simulink model "RCcasestudy"  (R2020a)
settings: Solver=VariableStepAuto  StartTime=0.0  StopTime=T  FixedStep=0  RelTol=1e-3
InitFcn:
  | run init.m
values from neighbouring files (symbols this model uses):
  C = 1e-2    (= 0.01)    [RCcasestudyscriptSample.m]    (also in init.m = 2e-06)
  C_1 = 2e-7    (= 2e-07)    [RCcasestudyscriptSample.m]    (also in init.m)
  C_2 = 2e-6    (= 2e-06)    [RCcasestudyscriptSample.m]    (also in init.m)
  R = 1000    [RCcasestudyscriptSample.m]    (also in init.m)
  R_1 = 320    [RCcasestudyscriptSample.m]    (also in init.m)
  R_2 = 400    [RCcasestudyscriptSample.m]    (also in init.m)
undefined symbols (not defined in the file or in its folder): Fs
libraries: slctrlblks x3
settings Model: Creator=ethan  LastModifiedBy=ethan
settings DataIOCC: ReturnWorkspaceOutputsName=simdata

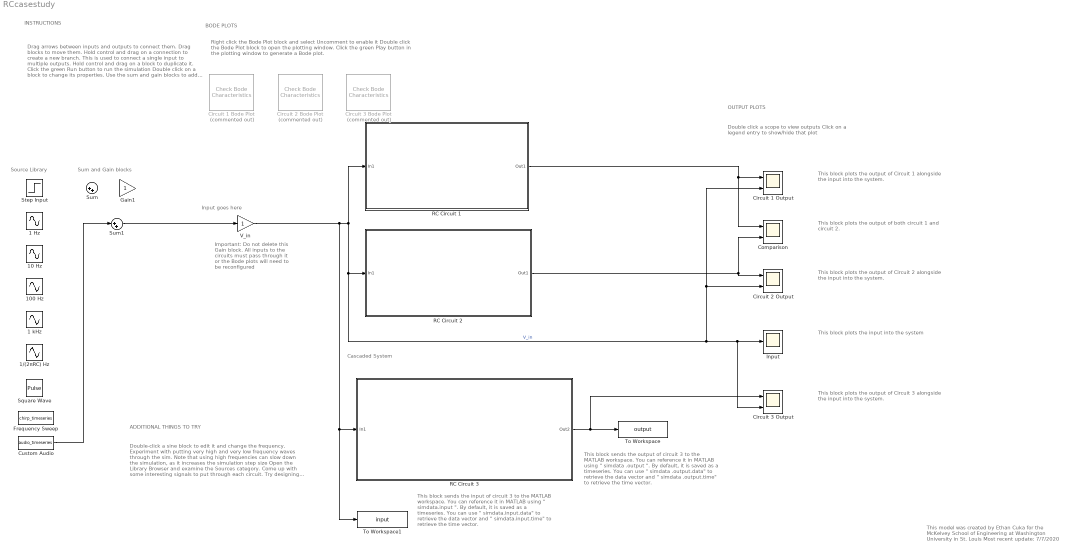
== system RCcasestudy ==
  note: This model was created by Ethan Cuka for the McKelvey School of Engineering at Washington University in St. Louis
      | Most recent update: 7/7/2020
  note: Double click a scope to view outputs
      |
      | Click on a legend entry to show/hide that plot
  note: Cascaded System
  note: Input goes here
  note: Sum and Gain blocks
  note: INSTRUCTIONS
  note: Source Library
  note: Important: Do not delete this Gain block. All inputs to the circuits must pass through it or the Bode plots will need to be reconfigured
  note: Right click the Bode Plot block and select Uncomment to enable it
      |
      | Double click the Bode Plot block to open the plotting window.
      |
      | Click the green Play button in the plotting window to generate a Bode plot.
  note: Drag arrows between inputs and outputs to connect them. Drag blocks to move them.
      |
      | Hold control and drag on a connection to create a new branch. This is used to connect a single input to multiple outputs. Hold control and drag on a block to duplicate it.
      |
      | Click the green Run button to run the simulation
      |
      | Double click on a block to change its properties.
      |
      | Use the sum and gain blocks to add combinations of waveforms together to create a superposition. Explore what happens to superimposed signals as they pass through each circuit.
  note: BODE PLOTS
  note: OUTPUT PLOTS
  note: This block plots the output of Circuit 1 alongside the input into the system.
  note: This block plots the output of both circuit 1 and circuit 2.
  note: This block plots the output of Circuit 2 alongside the input into the system.
  note: This block plots the input into the system
  note: This block plots the output of Circuit 3 alongside the input into the system.
  note: This block sends the output of circuit 3 to the MATLAB workspace. You can reference it in MATLAB using " simdata .output ". By default, it is saved as a timeseries. You can use " simdata .output.data" to retrieve the data vector and " simdata .output.time" to retrieve the time vector.
  note: ADDITIONAL THINGS TO TRY
  note: Double-click a sine block to edit it and change the frequency. Experiment with putting very high and very low frequency waves through the sim. Note that using high frequencies can slow down the simulation, as it increases the simulation step size
      |
      | Open the Library Browser and examine the Sources category. Come up with some interesting signals to put through each circuit.
      |
      | Try designing your own circuit to test. The simplest implementation in Simulink is to find the transfer function of your circuit and use the Transfer Function block.
  note: This block sends the input of circuit 3 to the MATLAB workspace. You can reference it in MATLAB using " simdata.input ". By default, it is saved as a timeseries. You can use " simdata.input.data" to retrieve the data vector and " simdata.input.time" to retrieve the time vector.
  1 Hz : Sin  Frequency=2*pi  SampleTime=0
  1 kHz : Sin  Frequency=2*pi*1000  SampleTime=0
  1/(2πRC) Hz : Sin  Frequency=1/(R*C)  SampleTime=0
  10 Hz : Sin  Frequency=2*pi*10  SampleTime=0
  100 Hz : Sin  Frequency=2*pi*100  SampleTime=0
  Circuit 1 Bode Plot : slctrlblks/Model Verification/Check Bode  Characteristics  Commented=on  InstantiateOnLoad=on  SaveOperatingPoints=off  LinearizationIOs={'/RC Circuit 1', 1, 'out', 'on', '';'/V_in', 1, 'in', 'off', ''}  LinearizeAt=SnapshotTimes  SnapshotTimes=[0]  TriggerType=rising  SampleTime=auto  RateConversionMethod=zoh  PreWarpFreq=10  UseExactDelayModel=off  UseFullBlockNameLabels=off  UseBusSignalLabels=off  enabled=on  stopWhenAssertionFail=off  export=off  ViewDlgPos=[-2.2 145 764.8 518.4]  OpenViewOnLoad=on  LaunchViewOnOpen=on  FrequencyUnits=rad/s  MagnitudeUnits=dB  PhaseUnits=deg  TimeUnits=seconds  EnableUpperBound=off  UpperBoundFrequencies=[]  UpperBoundMagnitudes=[]  EnableLowerBound=off  LowerBoundFrequencies=[]  LowerBoundMagnitudes=[]
      settings: SaveToWorkspace=on  SaveName=bode
  Circuit 1 Output : Scope  NumInputPorts=2
  Circuit 2 Bode Plot : slctrlblks/Model Verification/Check Bode  Characteristics  Commented=on  InstantiateOnLoad=on  SaveOperatingPoints=off  LinearizationIOs={'/RC Circuit 2', 1, 'out', 'on', '';'/V_in', 1, 'in', 'off', ''}  LinearizeAt=SnapshotTimes  SnapshotTimes=[0]  TriggerType=rising  SampleTime=auto  RateConversionMethod=zoh  PreWarpFreq=10  UseExactDelayModel=off  UseFullBlockNameLabels=off  UseBusSignalLabels=off  enabled=on  stopWhenAssertionFail=off  export=off  ViewDlgPos=[669.8 114.6 831.2 515.2]  OpenViewOnLoad=on  LaunchViewOnOpen=on  FrequencyUnits=rad/s  MagnitudeUnits=dB  PhaseUnits=deg  TimeUnits=seconds  EnableUpperBound=off  UpperBoundFrequencies=[]  UpperBoundMagnitudes=[]  EnableLowerBound=off  LowerBoundFrequencies=[]  LowerBoundMagnitudes=[]
  Circuit 2 Output : Scope  NumInputPorts=2
  Circuit 3 Bode Plot : slctrlblks/Model Verification/Check Bode  Characteristics  Commented=on  InstantiateOnLoad=on  SaveOperatingPoints=off  LinearizationIOs={'/RC Circuit 3', 1, 'out', 'on', '';'/V_in', 1, 'in', 'off', ''}  LinearizeAt=SnapshotTimes  SnapshotTimes=[0]  TriggerType=rising  SampleTime=auto  RateConversionMethod=zoh  PreWarpFreq=10  UseExactDelayModel=off  UseFullBlockNameLabels=off  UseBusSignalLabels=off  enabled=on  stopWhenAssertionFail=off  export=off  ViewDlgPos=[100 200 1266.6 390]  OpenViewOnLoad=off  LaunchViewOnOpen=on  FrequencyUnits=rad/s  MagnitudeUnits=dB  PhaseUnits=deg  TimeUnits=seconds  EnableUpperBound=off  UpperBoundFrequencies=[]  UpperBoundMagnitudes=[]  EnableLowerBound=off  LowerBoundFrequencies=[]  LowerBoundMagnitudes=[]
  Circuit 3 Output : Scope  NumInputPorts=2
  Comparison : Scope  NumInputPorts=2
  Custom Audio : FromWorkspace  VariableName=audio_timeseries  SampleTime=1/Fs
  Frequency Sweep : FromWorkspace  VariableName=chirp_timeseries  SampleTime=1/Fs
  Gain1 : Gain
  Input : Scope
  RC Circuit 1 : Subsystem
      mask Display: image(imread('circuit1.png'))
  RC Circuit 2 : Subsystem
      mask Display: image(imread('circuit2.png'))
  RC Circuit 3 : Subsystem
      mask Display: image(imread('circuit3.png'))
  Square Wave : DiscretePulseGenerator  PulseType=Time based  Period=.2  PulseWidth=50
  Step Input : Step  SampleTime=0
  Sum : Sum  Inputs=|++
  Sum1 : Sum  Inputs=|++
  To Workspace : ToWorkspace  VariableName=output  SaveFormat=Timeseries  SampleTime=-1
  To Workspace1 : ToWorkspace  VariableName=input  SaveFormat=Timeseries  SampleTime=-1
  V_in : Gain
  wires:
  RC Circuit 1/1(Out1) -> Circuit 1 Output/1, Comparison/1
  RC Circuit 2/1(Out1) -> Comparison/2, Circuit 2 Output/1
  RC Circuit 3/1(Out2) -> Circuit 3 Output/1, To Workspace/1
  V_in/1 -> To Workspace1/1, RC Circuit 3/1(In1), Circuit 3 Output/2, Input/1, Circuit 1 Output/2, Circuit 2 Output/2, RC Circuit 2/1(In1), RC Circuit 1/1(In1)  "V_in"
  Sum1/1 -> V_in/1
  Custom Audio/1 -> Sum1/1

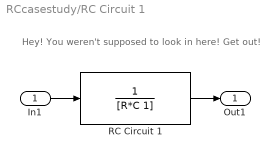
== system RCcasestudy/RC Circuit 1 ==
  note: Hey! You weren't supposed to look in here! Get out!
  In1 : Inport
  RC Circuit 1 : TransferFcn  Denominator=[R*C 1]
  Out1 : Outport
  wires:
  RC Circuit 1/1 -> Out1/1
  In1/1 -> RC Circuit 1/1

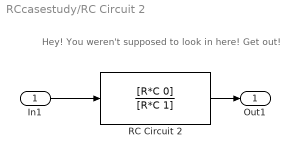
== system RCcasestudy/RC Circuit 2 ==
  note: Hey! You weren't supposed to look in here! Get out!
  In1 : Inport
  RC Circuit 2 : TransferFcn  Numerator=[R*C 0]  Denominator=[R*C 1]
  Out1 : Outport
  wires:
  RC Circuit 2/1 -> Out1/1
  In1/1 -> RC Circuit 2/1

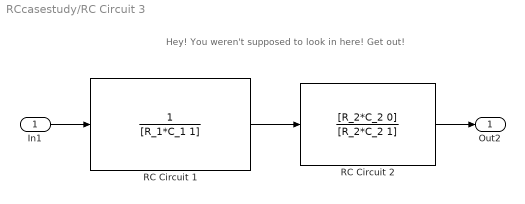
== system RCcasestudy/RC Circuit 3 ==
  note: Hey! You weren't supposed to look in here! Get out!
  In1 : Inport
  RC Circuit 1 : TransferFcn  Denominator=[R_1*C_1 1]
  RC Circuit 2 : TransferFcn  Numerator=[R_2*C_2 0]  Denominator=[R_2*C_2 1]
  Out2 : Outport
  wires:
  In1/1 -> RC Circuit 1/1
  RC Circuit 2/1 -> Out2/1
  RC Circuit 1/1 -> RC Circuit 2/1
